simulink model "second_order_system"  (R2020a)
settings: Solver=VariableStepAuto  StartTime=0.0  StopTime=10.0  RelTol=1e-3
undefined symbols (not defined in the file): wn, zeta
settings Model: Creator=Administrator  LastModifiedBy=Administrator

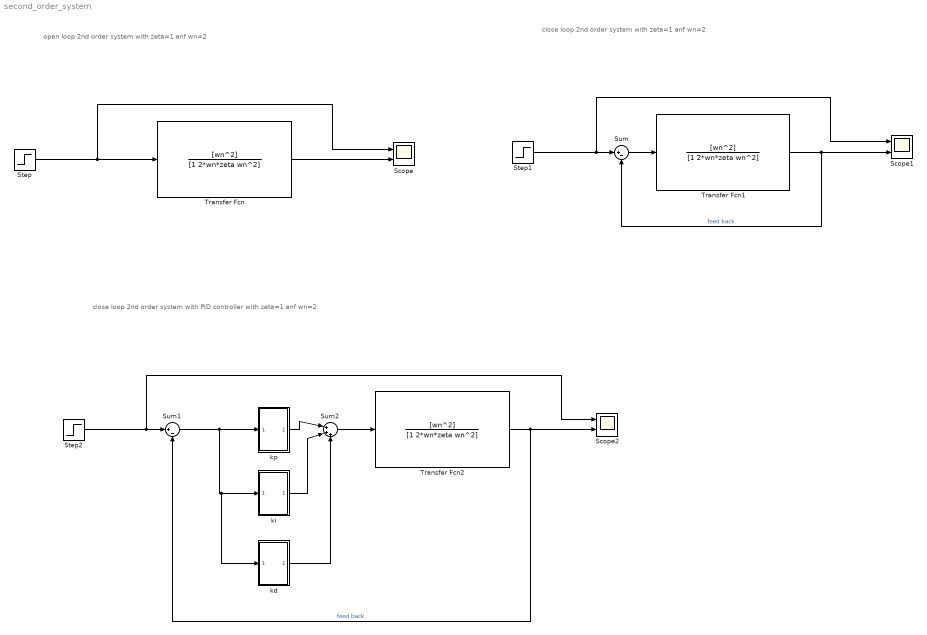
== system second_order_system ==
  note: open loop 2nd order system with zeta=1 anf wn=2
  note: close loop 2nd order system with zeta=1 anf wn=2
  note: close loop 2nd order system with PID controller with zeta=1 anf wn=2
  Scope : Scope  NumInputPorts=2
  Scope1 : Scope  NumInputPorts=2
  Scope2 : Scope  NumInputPorts=2
  Step : Step  SampleTime=0
  Step1 : Step  SampleTime=0
  Step2 : Step  SampleTime=0
  Sum : Sum  Inputs=|+-
  Sum1 : Sum  Inputs=|+-
  Sum2 : Sum  Inputs=|+++
  Transfer Fcn : TransferFcn  Numerator=[wn^2]  Denominator=[1 2*wn*zeta wn^2]
  Transfer Fcn1 : TransferFcn  Numerator=[wn^2]  Denominator=[1 2*wn*zeta wn^2]
  Transfer Fcn2 : TransferFcn  Numerator=[wn^2]  Denominator=[1 2*wn*zeta wn^2]
  kd : Subsystem
  ki : Subsystem
  kp : Subsystem
  wires:
  Step/1 -> Scope/1, Transfer Fcn/1
  Transfer Fcn/1 -> Scope/2
  Transfer Fcn1/1 -> Sum/2, Scope1/2  "feed back"
  Step1/1 -> Sum/1, Scope1/1
  Sum/1 -> Transfer Fcn1/1
  Sum1/1 -> kd/1(In1), ki/1(In1), kp/1(In1)
  Step2/1 -> Scope2/1, Sum1/1
  Transfer Fcn2/1 -> Sum1/2, Scope2/2  "feed back"
  kp/1(Out1) -> Sum2/1
  ki/1(Out1) -> Sum2/2
  Sum2/1 -> Transfer Fcn2/1
  kd/1(Out1) -> Sum2/3

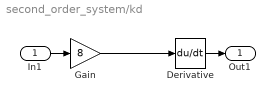
== system second_order_system/kd ==
  In1 : Inport
  Derivative : Derivative
  Gain : Gain  Gain=8
  Out1 : Outport
  wires:
  Derivative/1 -> Out1/1
  Gain/1 -> Derivative/1
  In1/1 -> Gain/1

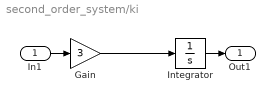
== system second_order_system/ki ==
  In1 : Inport
  Gain : Gain  Gain=3
  Integrator : Integrator
  Out1 : Outport
  wires:
  In1/1 -> Gain/1
  Gain/1 -> Integrator/1
  Integrator/1 -> Out1/1

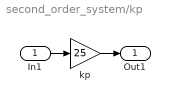
== system second_order_system/kp ==
  In1 : Inport
  kp : Gain  Gain=25
  Out1 : Outport
  wires:
  In1/1 -> kp/1
  kp/1 -> Out1/1
